simulink model "ex_54_j"  (R2018a)
settings: Solver=ode45  StartTime=0.0  StopTime=5  FixedStep=1e-5  RelTol=1e-5
values from neighbouring files (symbols this model uses):
  J = 0.5    [Ex54.m]
  L_s = L_ssig+L_sm    (= 0.085)    [Ex54.m]
  om_Ki = 24000    [Ex54.m]
  om_Kp = 320    [Ex54.m]
  omega_ref = 300    [Ex54.m]
  p = 1    [Ex54.m]
  psi_R0 = 1e-4    (= 0.0001)    [Ex54.m]
  R_R_m = (M/L_r)^2*R_r_m    [Ex54.m]
  rho_0 = 0    [Ex54.m]
  sigma = 1-M^2/L_s/L_r    [Ex54.m]
  t_l = 1.5    [Ex54.m]
  T_L = 50    [Ex54.m]
  tau_r = L_r/R_r    (= 0.141666666667)    [Ex54.m]
  tau_r_m = L_r/R_r_m    (= 0.0708333333333)    [Ex54.m]
  tau_u = 0.5e-3    (= 0.0005)    [Ex54.m]
settings Model: Creator=jianningdong  LastModifiedBy=Niels

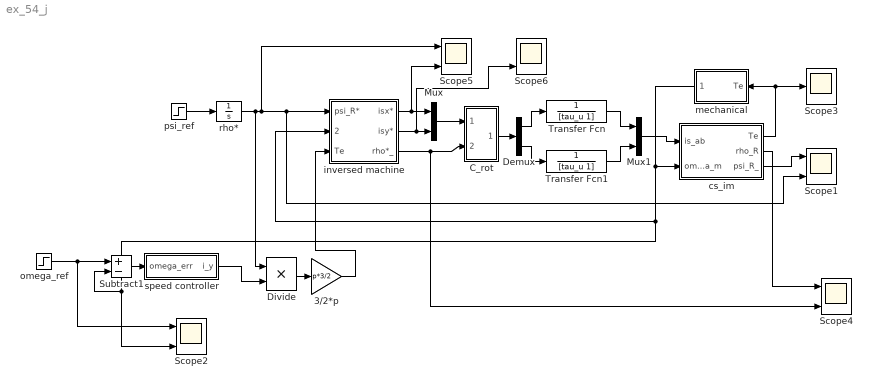
== system ex_54_j ==
  3/2*p : Gain  Gain=p*3/2  SaturateOnIntegerOverflow=on  OutDataTypeStr=Inherit: Same as input  ParamDataTypeStr=Inherit: Same as input
  C_rot : Subsystem
  Demux : Demux  Outputs=2
  Divide : Product  Inputs=**
  Mux : Mux  Inputs=2
  Mux1 : Mux  Inputs=2
  Scope{1..2,4..6} (5 alike) : Scope  NumInputPorts=2
  Scope3 : Scope
  Subtract1 : Sum  Inputs=+-
  Transfer Fcn : TransferFcn  Denominator=[tau_u 1]
  Transfer Fcn1 : TransferFcn  Denominator=[tau_u 1]
  cs_im : Subsystem
  inversed machine : Subsystem
  mechanical : Subsystem
  omega_ref : Step  Time=0.1  After=omega_ref  SampleTime=0
  psi_ref : Step  Time=0.01  After=31  SampleTime=0
  rho* : Integrator  InitialCondition=psi_R0  LimitOutput=on  UpperSaturationLimit=0.816
  speed controller : Subsystem
  wires:
  cs_im/1(Te) -> Scope3/1, mechanical/1(Te)
  mechanical/1(omega) -> cs_im/2(omega_m), inversed machine/2(omega_m), Scope2/2, Subtract1/2
  Mux/1 -> C_rot/1(in_1)
  C_rot/1(out_1) -> Demux/1
  Demux/1 -> Transfer Fcn/1
  Demux/2 -> Transfer Fcn1/1
  Transfer Fcn/1 -> Mux1/1
  Transfer Fcn1/1 -> Mux1/2
  Mux1/1 -> cs_im/1(is_ab)
  omega_ref/1 -> Scope2/1, Subtract1/1
  Subtract1/1 -> speed controller/1(omega_err)
  psi_ref/1 -> rho*/1
  inversed machine/1(isx*) -> Scope5/2, Mux/1
  inversed machine/2(isy*) -> Scope6/2, Mux/2
  inversed machine/3(rho*_) -> Scope4/2, C_rot/2(in_2)
  cs_im/3(psi_R_) -> Scope1/1
  cs_im/2(rho_R) -> Scope4/1
  rho*/1 -> Divide/1, Scope5/1, Scope1/2, inversed machine/1(psi_R*)
  speed controller/1(i_y) -> Divide/2
  Divide/1 -> 3/2*p/1
  3/2*p/1 -> inversed machine/3(Te)

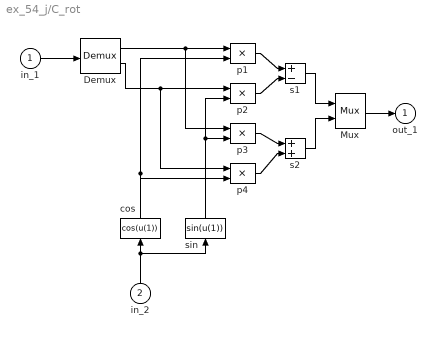
== system ex_54_j/C_rot ==
  in_1 : Inport
  in_2 : Inport  Port=2
  Demux : Demux  Outputs=2
  Mux : Mux  Inputs=2
  cos : Fcn  Expr=cos(u(1))
  p{1..4} (4 alike) : Product  SaturateOnIntegerOverflow=on  RndMeth=Zero  InputSameDT=on  OutDataTypeStr=Inherit: Same as first input
  s1 : Sum  Inputs=+-  SaturateOnIntegerOverflow=on  InputSameDT=on  OutDataTypeStr=Inherit: Same as first input
  s2 : Sum  SaturateOnIntegerOverflow=on  InputSameDT=on  OutDataTypeStr=Inherit: Same as first input
  sin : Fcn  Expr=sin(u(1))
  out_1 : Outport
  wires:
  s2/1 -> Mux/2
  s1/1 -> Mux/1
  p2/1 -> s1/2
  p3/1 -> s2/1
  p1/1 -> s1/1
  p4/1 -> s2/2
  in_2/1 -> cos/1, sin/1
  sin/1 -> p2/2, p3/2
  cos/1 -> p1/2, p4/2
  Demux/1 -> p1/1, p3/1
  Demux/2 -> p2/1, p4/1
  in_1/1 -> Demux/1
  Mux/1 -> out_1/1

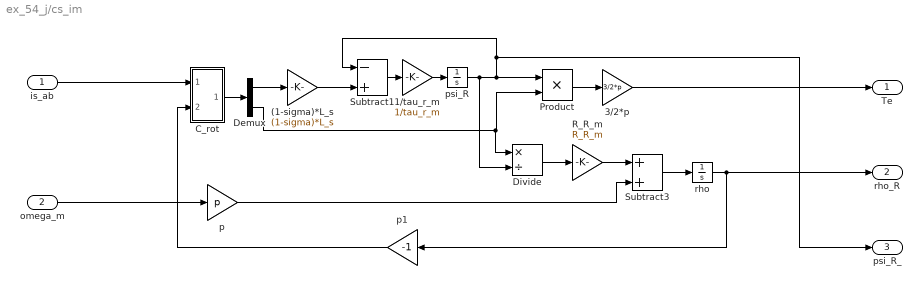
== system ex_54_j/cs_im ==
  is_ab : Inport
  omega_m : Inport  Port=2
  (1-sigma)*L_s : Gain  Gain=(1-sigma)*L_s  SaturateOnIntegerOverflow=on  OutDataTypeStr=Inherit: Same as input  ParamDataTypeStr=Inherit: Same as input
  1/tau_r_m : Gain  Gain=1/tau_r_m  SaturateOnIntegerOverflow=on  OutDataTypeStr=Inherit: Same as input  ParamDataTypeStr=Inherit: Same as input
  3/2*p : Gain  Gain=3/2*p  SaturateOnIntegerOverflow=on  OutDataTypeStr=Inherit: Same as input  ParamDataTypeStr=Inherit: Same as input
  C_rot : Subsystem
  Demux : Demux  Outputs=2
  Divide : Product  Inputs=*/
  Product : Product
  R_R_m : Gain  Gain=R_R_m  SaturateOnIntegerOverflow=on  OutDataTypeStr=Inherit: Same as input  ParamDataTypeStr=Inherit: Same as input
  Subtract1 : Sum  Inputs=-+
  Subtract3 : Sum
  p : Gain  Gain=p  SaturateOnIntegerOverflow=on  OutDataTypeStr=Inherit: Same as input  ParamDataTypeStr=Inherit: Same as input
  p1 : Gain  Gain=-1  SaturateOnIntegerOverflow=on  OutDataTypeStr=Inherit: Same as input  ParamDataTypeStr=Inherit: Same as input
  psi_R : Integrator  InitialCondition=psi_R0
  rho : Integrator  InitialCondition=rho_0
  Te : Outport
  rho_R : Outport  Port=2
  psi_R_ : Outport  Port=3
  wires:
  C_rot/1(out_1) -> Demux/1
  Demux/2 -> Divide/1, Product/2
  (1-sigma)*L_s/1 -> Subtract1/2
  R_R_m/1 -> Subtract3/1
  Demux/1 -> (1-sigma)*L_s/1
  omega_m/1 -> p/1
  1/tau_r_m/1 -> psi_R/1
  3/2*p/1 -> Te/1
  Product/1 -> 3/2*p/1
  Subtract3/1 -> rho/1
  rho/1 -> rho_R/1, p1/1
  p/1 -> Subtract3/2
  Subtract1/1 -> 1/tau_r_m/1
  psi_R/1 -> Divide/2, Product/1, psi_R_/1, Subtract1/1
  is_ab/1 -> C_rot/1(in_1)
  Divide/1 -> R_R_m/1
  p1/1 -> C_rot/2(in_2)

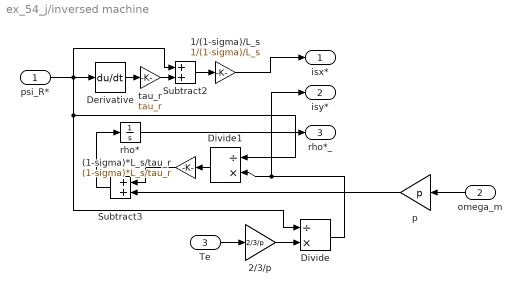
== system ex_54_j/inversed machine ==
  psi_R* : Inport
  omega_m : Inport  Port=2
  Te : Inport  Port=3
  (1-sigma)*L_s/tau_r : Gain  Gain=(1-sigma)*L_s/tau_r  SaturateOnIntegerOverflow=on  OutDataTypeStr=Inherit: Same as input  ParamDataTypeStr=Inherit: Same as input
  1/(1-sigma)/L_s : Gain  Gain=1/(1-sigma)/L_s  SaturateOnIntegerOverflow=on  OutDataTypeStr=Inherit: Same as input  ParamDataTypeStr=Inherit: Same as input
  2/3/p : Gain  Gain=2/3/p  SaturateOnIntegerOverflow=on  OutDataTypeStr=Inherit: Same as input  ParamDataTypeStr=Inherit: Same as input
  Derivative : Derivative
  Divide : Product  Inputs=/*
  Divide1 : Product  Inputs=/*
  Subtract2 : Sum
  Subtract3 : Sum
  p : Gain  Gain=p  SaturateOnIntegerOverflow=on  OutDataTypeStr=Inherit: Same as input  ParamDataTypeStr=Inherit: Same as input
  rho* : Integrator
  tau_r : Gain  Gain=tau_r  SaturateOnIntegerOverflow=on  OutDataTypeStr=Inherit: Same as input  ParamDataTypeStr=Inherit: Same as input
  isx* : Outport
  isy* : Outport  Port=2
  rho*_ : Outport  Port=3
  wires:
  omega_m/1 -> p/1
  Derivative/1 -> tau_r/1
  1/(1-sigma)/L_s/1 -> isx*/1
  Divide1/1 -> (1-sigma)*L_s/tau_r/1
  psi_R*/1 -> Divide1/1, Divide/1, Subtract2/1, Derivative/1
  tau_r/1 -> Subtract2/2
  Divide/1 -> isy*/1, Divide1/2
  Te/1 -> 2/3/p/1
  2/3/p/1 -> Divide/2
  Subtract2/1 -> 1/(1-sigma)/L_s/1
  p/1 -> Subtract3/2
  (1-sigma)*L_s/tau_r/1 -> Subtract3/1
  Subtract3/1 -> rho*/1
  rho*/1 -> rho*_/1

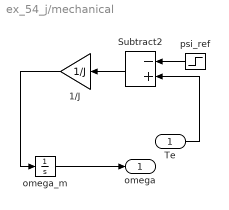
== system ex_54_j/mechanical ==
  Te : Inport
  1/J : Gain  Gain=1/J  SaturateOnIntegerOverflow=on  OutDataTypeStr=Inherit: Same as input  ParamDataTypeStr=Inherit: Same as input
  Subtract2 : Sum  Inputs=-+
  omega_m : Integrator
  psi_ref : Step  Time=t_l  After=T_L  SampleTime=0
  omega : Outport
  wires:
  Te/1 -> Subtract2/2
  Subtract2/1 -> 1/J/1
  1/J/1 -> omega_m/1
  omega_m/1 -> omega/1
  psi_ref/1 -> Subtract2/1

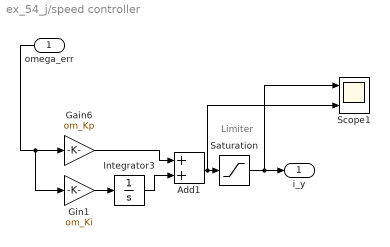
== system ex_54_j/speed controller ==
  note: Limiter
  omega_err : Inport
  Add1 : Sum
  Gain6 : Gain  Gain=om_Kp
  Gin1 : Gain  Gain=om_Ki
  Integrator3 : Integrator  LimitOutput=on  UpperSaturationLimit=122.5  LowerSaturationLimit=-122.5
  Saturation : Saturate  UpperLimit=122.5  LowerLimit=-122.5  ZeroCross=off
  Scope1 : Scope  NumInputPorts=2
  i_y : Outport
  wires:
  Integrator3/1 -> Add1/2
  Gin1/1 -> Integrator3/1
  Add1/1 -> Scope1/2, Saturation/1
  Gain6/1 -> Add1/1
  Saturation/1 -> Scope1/1, i_y/1
  omega_err/1 -> Gin1/1, Gain6/1

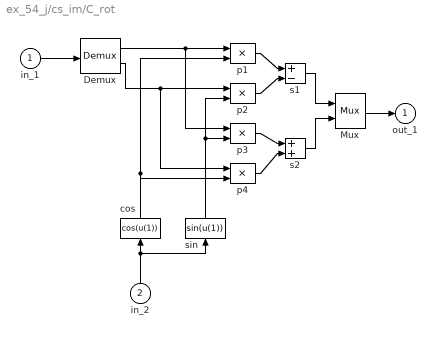
== system ex_54_j/cs_im/C_rot ==
  in_1 : Inport
  in_2 : Inport  Port=2
  Demux : Demux  Outputs=2
  Mux : Mux  Inputs=2
  cos : Fcn  Expr=cos(u(1))
  p{1..4} (4 alike) : Product  SaturateOnIntegerOverflow=on  RndMeth=Zero  InputSameDT=on  OutDataTypeStr=Inherit: Same as first input
  s1 : Sum  Inputs=+-  SaturateOnIntegerOverflow=on  InputSameDT=on  OutDataTypeStr=Inherit: Same as first input
  s2 : Sum  SaturateOnIntegerOverflow=on  InputSameDT=on  OutDataTypeStr=Inherit: Same as first input
  sin : Fcn  Expr=sin(u(1))
  out_1 : Outport
  wires:
  s2/1 -> Mux/2
  s1/1 -> Mux/1
  p2/1 -> s1/2
  p3/1 -> s2/1
  p1/1 -> s1/1
  p4/1 -> s2/2
  in_2/1 -> cos/1, sin/1
  sin/1 -> p2/2, p3/2
  cos/1 -> p1/2, p4/2
  Demux/1 -> p1/1, p3/1
  Demux/2 -> p2/1, p4/1
  in_1/1 -> Demux/1
  Mux/1 -> out_1/1
